simulink model "InvK_Decoupling_Approach_G18"  (R2016a)
settings: Solver=VariableStepAuto  SolverMode=SingleTasking  StartTime=0.0  StopTime=inf  RelTol=1e-3
libraries: vrlib x7, simulink_extras x6
settings Model: Creator=Ricardo Henriques  LastModifiedBy=Ricardo Henriques
settings DebuggingCC: SFUnexpectedBacktrackingDiag=error  SFNoUnconditionalDefaultTransitionDiag=error
settings GRTTargetCC: TargetLangStandard=C99 (ISO)  GeneratePreprocessorConditionals=Use local settings
settings ConfigComp: CovMetricSettings=dwe  CovHtmlReporting=off  CovSaveCumulativeToWorkspaceVar=off  CovSaveSingleToWorkspaceVar=off  CovExternalEMLEnable=on

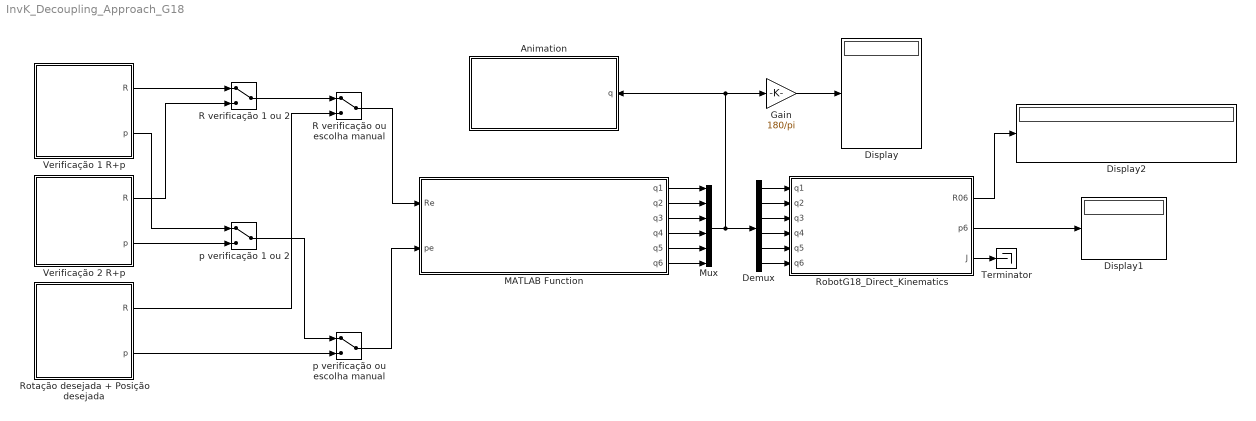
== system InvK_Decoupling_Approach_G18 ==
  "Animation " : Subsystem
  Demux : Demux  Outputs=6
  Display : Display
  Display1 : Display
  Display2 : Display
  Gain : Gain  Gain=180/pi
  MATLAB Function : MATLAB Function  TreatAsAtomicUnit=on
  Mux : Mux  Inputs=6
  R verificação 1 ou 2 : ManualSwitch
  R verificação ou escolha manual : ManualSwitch
  RobotG18_Direct_Kinematics : MATLAB Function  TreatAsAtomicUnit=on
  Rotação desejada + Posição desejada : Subsystem  mask{px=0.663, py=-0.109, pz=0.051, phi=0, theta=-180.0, psi=90}
  Terminator : Terminator
  Verificação 1 R+p : Subsystem
  Verificação 2 R+p : Subsystem
  p verificação 1 ou 2 : ManualSwitch
  p verificação ou escolha manual : ManualSwitch
  wires:
  MATLAB Function/1(q1) -> Mux/1
  MATLAB Function/2(q2) -> Mux/2
  MATLAB Function/6(q6) -> Mux/6
  MATLAB Function/5(q5) -> Mux/5
  MATLAB Function/4(q4) -> Mux/4
  MATLAB Function/3(q3) -> Mux/3
  Mux/1 -> "Animation "/1("q "), Gain/1, Demux/1
  Demux/1 -> RobotG18_Direct_Kinematics/1(q1)
  Demux/2 -> RobotG18_Direct_Kinematics/2(q2)
  Demux/3 -> RobotG18_Direct_Kinematics/3(q3)
  Demux/4 -> RobotG18_Direct_Kinematics/4(q4)
  Demux/5 -> RobotG18_Direct_Kinematics/5(q5)
  Demux/6 -> RobotG18_Direct_Kinematics/6(q6)
  RobotG18_Direct_Kinematics/3(J) -> Terminator/1
  RobotG18_Direct_Kinematics/2(p6) -> Display1/1
  RobotG18_Direct_Kinematics/1(R06) -> Display2/1
  Gain/1 -> Display/1
  R verificação ou escolha manual/1 -> MATLAB Function/1(Re)
  p verificação ou escolha manual/1 -> MATLAB Function/2(pe)
  R verificação 1 ou 2/1 -> R verificação ou escolha manual/1
  p verificação 1 ou 2/1 -> p verificação ou escolha manual/1
  Rotação desejada + Posição desejada/1(R) -> R verificação ou escolha manual/2
  Rotação desejada + Posição desejada/2(p) -> p verificação ou escolha manual/2
  Verificação 1 R+p/1(R) -> R verificação 1 ou 2/1
  Verificação 2 R+p/1(R) -> R verificação 1 ou 2/2
  Verificação 2 R+p/2(p) -> p verificação 1 ou 2/2
  Verificação 1 R+p/2(p) -> p verificação 1 ou 2/1

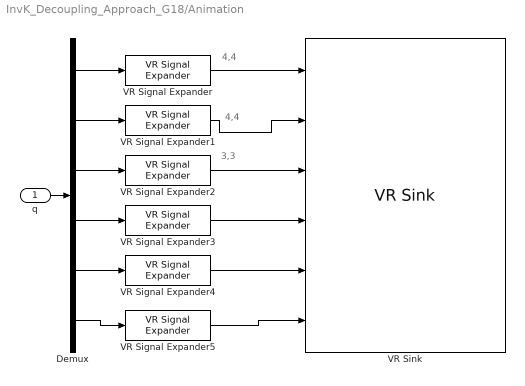
== system InvK_Decoupling_Approach_G18/Animation  ==
  note: 4,4
  note: 3,3
  note: 4,4
  "q " : Inport
  Demux : Demux  Outputs=6
  VR Signal Expander{,1..5} (6 alike) : vrlib/VR Signal Expander  outwidth=4  outidx=4
  VR Sink : vrlib/VR Sink  InstantiateOnLoad=on  SampleTime=0.1  ViewEnable=on  RemoteChange=off  RemoteView=off  FieldsWritten=Jt1_DH_dv.rotation.4.1.1.double#Jt2_DH_dv.rotation.4.1.1.double#Jt3_DH_dv.rotation.4.1.1.double#Jt4_DH_dv.rotation.4.1.1.double#Jt5_DH_dv.rotation.4.1.1.double#Jt6_DH_dv.rotation.4.1.1.double  WorldFileName=RobotG18_Opt_NoAxes.wrl  WorldDescription=D-H Reference Frames for Virtual Reality Robot  AutoView=off  VideoDimensions=[]  AllowVariableSize=off
  wires:
  "q "/1 -> Demux/1
  Demux/1 -> VR Signal Expander/1
  Demux/2 -> VR Signal Expander1/1
  Demux/3 -> VR Signal Expander2/1
  Demux/4 -> VR Signal Expander3/1
  Demux/5 -> VR Signal Expander4/1
  Demux/6 -> VR Signal Expander5/1
  VR Signal Expander/1 -> VR Sink/1
  VR Signal Expander1/1 -> VR Sink/2
  VR Signal Expander5/1 -> VR Sink/6
  VR Signal Expander2/1 -> VR Sink/3
  VR Signal Expander3/1 -> VR Sink/4
  VR Signal Expander4/1 -> VR Sink/5

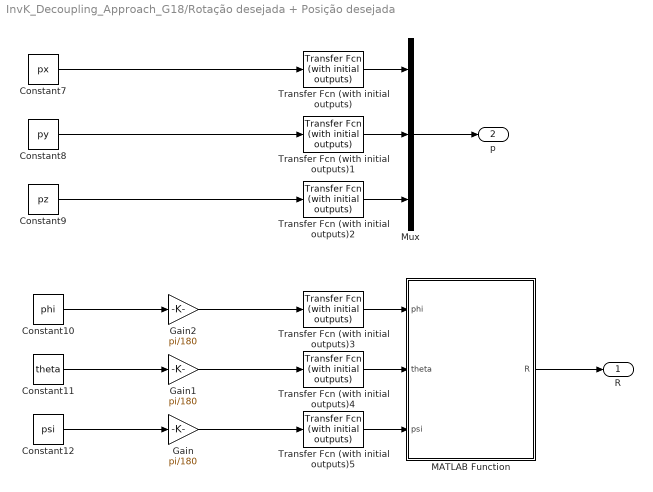
== system InvK_Decoupling_Approach_G18/Rotação desejada + Posição desejada ==
  Constant10 : Constant  Value=phi
  Constant11 : Constant  Value=theta
  Constant12 : Constant  Value=psi
  Constant7 : Constant  Value=px
  Constant8 : Constant  Value=py
  Constant9 : Constant  Value=pz
  Gain : Gain  Gain=pi/180
  Gain1 : Gain  Gain=pi/180
  Gain2 : Gain  Gain=pi/180
  MATLAB Function : MATLAB Function  TreatAsAtomicUnit=on
  Mux : Mux  Inputs=3
  Transfer Fcn (with initial outputs) : simulink_extras/Additional Linear/Transfer Fcn (with initial outputs)  N=[2]  D="[1  2]"  Y0=px  U0=0
  Transfer Fcn (with initial outputs)1 : simulink_extras/Additional Linear/Transfer Fcn (with initial outputs)  N=[2]  D="[1  2]"  Y0=py  U0=0
  Transfer Fcn (with initial outputs)2 : simulink_extras/Additional Linear/Transfer Fcn (with initial outputs)  N=[2]  D="[1  2]"  Y0=pz  U0=0
  Transfer Fcn (with initial outputs)3 : simulink_extras/Additional Linear/Transfer Fcn (with initial outputs)  N=[2]  D="[1  2]"  Y0=phi  U0=0
  Transfer Fcn (with initial outputs)4 : simulink_extras/Additional Linear/Transfer Fcn (with initial outputs)  N=[2]  D="[1  2]"  Y0=theta  U0=0
  Transfer Fcn (with initial outputs)5 : simulink_extras/Additional Linear/Transfer Fcn (with initial outputs)  N=[2]  D="[1  2]"  Y0=psi  U0=0
  R : Outport
  p : Outport  Port=2
  wires:
  Constant8/1 -> Transfer Fcn (with initial outputs)1/1
  Constant9/1 -> Transfer Fcn (with initial outputs)2/1
  Constant12/1 -> Gain/1
  Constant7/1 -> Transfer Fcn (with initial outputs)/1
  Constant11/1 -> Gain1/1
  Constant10/1 -> Gain2/1
  Transfer Fcn (with initial outputs)5/1 -> MATLAB Function/3(psi)
  Transfer Fcn (with initial outputs)3/1 -> MATLAB Function/1(phi)
  Transfer Fcn (with initial outputs)4/1 -> MATLAB Function/2(theta)
  Transfer Fcn (with initial outputs)/1 -> Mux/1
  Transfer Fcn (with initial outputs)1/1 -> Mux/2
  Transfer Fcn (with initial outputs)2/1 -> Mux/3
  Gain2/1 -> Transfer Fcn (with initial outputs)3/1
  Gain1/1 -> Transfer Fcn (with initial outputs)4/1
  Gain/1 -> Transfer Fcn (with initial outputs)5/1
  Mux/1 -> p/1
  MATLAB Function/1(R) -> R/1

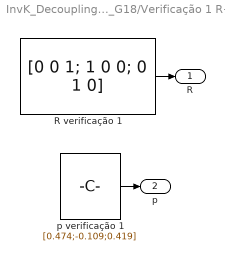
== system InvK_Decoupling_Approach_G18/Verificação 1 R+p ==
  R verificação 1 : Constant  Value=[0 0 1; 1 0 0; 0 1 0]  VectorParams1D=off
  p verificação 1 : Constant  Value=[0.474;-0.109;0.419]  VectorParams1D=off
  R : Outport
  p : Outport  Port=2
  wires:
  p verificação 1/1 -> p/1
  R verificação 1/1 -> R/1

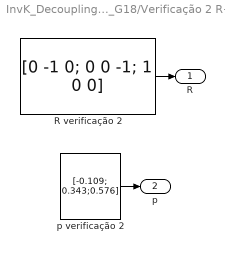
== system InvK_Decoupling_Approach_G18/Verificação 2 R+p ==
  R verificação 2 : Constant  Value=[0 -1 0; 0 0 -1; 1 0 0]  VectorParams1D=off
  p verificação 2 : Constant  Value=[-0.109; 0.343;0.576]  VectorParams1D=off
  R : Outport
  p : Outport  Port=2
  wires:
  p verificação 2/1 -> p/1
  R verificação 2/1 -> R/1

== matlab function InvK_Decoupling_Approach_G18/RobotG18_Direct_Kinematics ==
  data: q1 input; R06 output; q2 input; q3 input; q4 input; q5 input; q6 input; p6 output; J output
function [R06,p6,J] = RobotG18_Direct_Kinematics(q1,q2,q3,q4,q5,q6)
%#codegen

%    This function was generated by the Symbolic Math Toolbox version 7.0.
%    15-Apr-2021 18:49:51

t2 = q2+q3+q4;
t3 = cos(q1);
t4 = sin(q6);
t5 = sin(q1);
t6 = sin(q5);
t7 = t5.*t6;
t8 = cos(t2);
t9 = cos(q5);
t10 = t7-t3.*t8.*t9;
t11 = sin(t2);
t12 = cos(q6);
t13 = t3.*t6;
t14 = t5.*t8.*t9;
t15 = t13+t14;
t16 = q2+q3;
t17 = cos(q2);
t18 = sin(q2);
t19 = sin(q3);
t20 = cos(t16);
t21 = sin(q4);
t22 = sin(t16);
t23 = cos(q4);
t24 = cos(q3);
t25 = t5.*t17.*(1.7e1./4.0e1);
t26 = t5.*t6.*t8.*(4.1e1./5.0e2);
t27 = t5.*t17.*t24.*(4.9e1./1.25e2);
t28 = t22.*(4.9e1./1.25e2);
t29 = t18.*(1.7e1./4.0e1);
t30 = t20.*t21.*(4.1e1./5.0e2);
t31 = t22.*t23.*(4.1e1./5.0e2);
t32 = t30+t31;
t33 = t6.*t32;
t34 = t20.*t23.*(1.9e1./2.0e2);
t35 = t8.*(1.9e1./2.0e2);
t36 = t6.*t11.*(4.1e1./5.0e2);
t37 = t5.*(1.09e2./1.0e3);
t38 = t3.*t17.*(1.7e1./4.0e1);
t39 = t5.*t9.*(4.1e1./5.0e2);
t40 = t3.*t6.*t8.*(4.1e1./5.0e2);
t41 = t3.*t17.*t24.*(4.9e1./1.25e2);
t42 = t37+t38+t39+t40+t41-t3.*t18.*t19.*(4.9e1./1.25e2)-t3.*t20.*t21.*(1.9e1./2.0e2)-t3.*t22.*t23.*(1.9e1./2.0e2);
t43 = t28+t29+t33+t34-t21.*t22.*(1.9e1./2.0e2);
t44 = t28+t35+t36;
t45 = t35+t36;
t46 = q2+q3+q4+q5;
t47 = sin(t46);
t48 = t47.*(4.1e1./1.0e3);
t49 = t20.*(4.9e1./1.25e2);
t50 = q2+q3+q4-q5;
t51 = sin(t50);
t52 = t5.*t9;
t53 = t3.*t6.*t8;
t54 = t52+t53;
t55 = t5.*t6.*t8;
t56 = t55-t3.*t9;
t57 = t6.*t11;
R06 = reshape([-t10.*t12-t3.*t4.*t11,t12.*t15-t4.*t5.*t11,t4.*t8+t9.*t11.*t12,t4.*t10-t3.*t11.*t12,-t4.*t15-t5.*t11.*t12,t8.*t12-t4.*t9.*t11,t54,t56,t57],[3,3]);
if nargout > 1
    p6 = [t42;t3.*(-1.09e2./1.0e3)+t25+t26+t27-t3.*t9.*(4.1e1./5.0e2)-t5.*t18.*t19.*(4.9e1./1.25e2)-t5.*t20.*t21.*(1.9e1./2.0e2)-t5.*t22.*t23.*(1.9e1./2.0e2);t28+t29+t33+t34-t21.*t22.*(1.9e1./2.0e2)+8.9e1./1.0e3];
end
if nargout > 2
    J = reshape([t3.*(1.09e2./1.0e3)-t25-t26-t27+t3.*t9.*(4.1e1./5.0e2)+t5.*t18.*t19.*(4.9e1./1.25e2)+t5.*t20.*t21.*(1.9e1./2.0e2)+t5.*t22.*t23.*(1.9e1./2.0e2),t42,0.0,0.0,0.0,1.0,-t3.*t43,-t5.*t43,t11.*(-1.9e1./2.0e2)+t17.*(1.7e1./4.0e1)+t48+t49-t51.*(4.1e1./1.0e3),t5,-t3,0.0,-t3.*t44,-t5.*t44,t11.*(-1.9e1./2.0e2)+t48+t49-t51.*(4.1e1./1.0e3),t5,-t3,0.0,-t3.*t45,-t5.*t45,t11.*(-1.9e1./2.0e2)+t48-t51.*(4.1e1./1.0e3),t5,-t3,0.0,t5.*t6.*(-4.1e1./5.0e2)-t3.*t9.*t17.*t19.*t21.*(4.1e1./5.0e2)-t3.*t9.*t18.*t19.*t23.*(4.1e1./5.0e2)-t3.*t9.*t18.*t21.*t24.*(4.1e1./5.0e2)+t3.*t9.*t17.*t23.*t24.*(4.1e1./5.0e2),t3.*t6.*(4.1e1./5.0e2)-t5.*t9.*t17.*t19.*t21.*(4.1e1./5.0e2)-t5.*t9.*t18.*t19.*t23.*(4.1e1./5.0e2)-t5.*t9.*t18.*t21.*t24.*(4.1e1./5.0e2)+t5.*t9.*t17.*t23.*t24.*(4.1e1./5.0e2),t48+t51.*(4.1e1./1.0e3),-t3.*t11,-t5.*t11,t8,0.0,0.0,0.0,t54,t56,t57],[6,6]);
end

== matlab function InvK_Decoupling_Approach_G18/MATLAB Function ==
  data: Re input; q1 output; pe input; q2 output; q3 output; q4 output; q5 output; q6 output
function [q1,q2,q3,q4,q5,q6] = Robot618_Inverse_Kinematics_Decoupling(Re,pe)
% Esta função cálcula os ângulos das juntas de rotação através da abordagem
% do desacoplamento.
%
% Inputs: - Re: Matriz de Rotação entre o referêncial 6 e o referencial 0.
%         - pe: Vetor de posição do referêncial 6 em relação ao referencial 0
%
% Outputs: - q1,q2,q3,q4,q5,q6: ângulos entre os eixos x_i-1 e x_i sobre o
% eixo z_i.
%
% Catarina Pires 90230
% Ricardo Henriques 90349
% Última Edição: 22/04/2021
% ------------------------------------------------------------------------
%Cálculo da Matriz de Transformação Homogénea
A06_v = zeros(4,4);
A06_v(1:3,1:3) = Re;
A06_v(1:3,4) = pe;
A06_v(4,4) = 1;
d4 = 0.109;
d6 = 0.082;
a2 = 0.425;
a3 = 0.392;

%Cálculo q1
P05 = A06_v*[0;0;-d6;1] - [0;0;0;1];
P05_xy = sqrt(P05(1).^2 + P05(2).^2);
if pe(2,1)>0
    fi = acos(d4/P05_xy);          %verificar o quadrante 
elseif pe(2,1)==0
    if pe(1,1)<0
        fi = -acos(d4/P05_xy);
    else
        fi = acos(d4/P05_xy);
    end
else
    fi = -acos(d4/P05_xy);
end
qsi = atan2(P05(2),P05(1));
q1 = fi + qsi + pi/2;

%Cálculo q5
P16_z = pe(1)*sin(q1) - pe(2)*cos(q1);

if Re(3,1)>0 && Re(3,1)<=1
    q5 = acos((P16_z - d4)/d6);     %verificar o quadrante 
else
    q5 = -acos((P16_z - d4)/d6);
end

%Cálculo q6
DH_6 = [ 0.089    q1    0    pi/2    0; %    'R';
    0        0  0.425    0     0; %    'R';
    0        0  0.392    0     0; %    'R';
    0.109    0    0   -pi/2    0; %    'R';
    0.095    q5    0    pi/2    0; %    'R';
    0.082    0    0     0      0];%    'R'];
p = DH_6(1,1:5);
A01 =[cos(p(2)) -sin(p(2))*cos(p(4))  sin(p(2))*sin(p(4)) p(3)*cos(p(2));
    sin(p(2))  cos(p(2))*cos(p(4)) -cos(p(2))*sin(p(4)) p(3)*sin(p(2));
    0          sin(p(4))            cos(p(4))                 p(1)    ;
    0             0                    0                        1     ];
A61 = inv(inv(A01)*A06_v);
R61= A61(1:3,1:3);
q6 = atan2(R61(2,3),R61(1,3));

%Cálculo q3
DH_3 = [ 0.089    q1    0    pi/2    0; %    'R';
    0        0  0.425    0     0; %    'R';
    0        0  0.392    0     0; %    'R';
    0.109    0    0   -pi/2    0; %    'R';
    0.095    q5    0    pi/2    0; %    'R';
    0.082    q6    0     0      0];%    'R'];
p = DH_3(5,1:5);
A45 =[cos(p(2)) -sin(p(2))*cos(p(4))  sin(p(2))*sin(p(4)) p(3)*cos(p(2));
    sin(p(2))  cos(p(2))*cos(p(4)) -cos(p(2))*sin(p(4)) p(3)*sin(p(2));
    0          sin(p(4))            cos(p(4))                 p(1)    ;
    0             0                    0                        1     ];
p = DH_3(6,1:5);
A56 =[cos(p(2)) -sin(p(2))*cos(p(4))  sin(p(2))*sin(p(4)) p(3)*cos(p(2));
    sin(p(2))  cos(p(2))*cos(p(4)) -cos(p(2))*sin(p(4)) p(3)*sin(p(2));
    0          sin(p(4))            cos(p(4))                 p(1)    ;
    0             0                    0                        1     ];
A14 = inv(A61)*inv(A45*A56);
P13 = A14*[0;d4;0;1] - [0;0;0;1];
q3 = -acos((norm(P13).^2 - a2^2 - a3^2)/(2*a2*a3));

%Cálculo q2
q2 = atan2(P13(2),(P13(1))) - asin((a3*sin(q3)/norm(P13)));

%Cálculo q4
DH_4 = [ 0.089    q1    0    pi/2    0; %    'R';
    0       q2  0.425    0     0; %    'R';
    0       q3  0.392    0     0; %    'R';
    0.109    0    0   -pi/2    0; %    'R';
    0.095    q5    0    pi/2    0; %    'R';
    0.082    q6    0     0      0];%    'R'];
p = DH_4(2,1:5);
A12 =[cos(p(2)) -sin(p(2))*cos(p(4))  sin(p(2))*sin(p(4)) p(3)*cos(p(2));
    sin(p(2))  cos(p(2))*cos(p(4)) -cos(p(2))*sin(p(4)) p(3)*sin(p(2));
    0          sin(p(4))            cos(p(4))                 p(1)    ;
    0             0                    0                        1     ];
p = DH_4(3,1:5);
A23 =[cos(p(2)) -sin(p(2))*cos(p(4))  sin(p(2))*sin(p(4)) p(3)*cos(p(2));
    sin(p(2))  cos(p(2))*cos(p(4)) -cos(p(2))*sin(p(4)) p(3)*sin(p(2));
    0          sin(p(4))            cos(p(4))                 p(1)    ;
    0             0                    0                        1     ];
A34 = inv(A12*A23)*A14;
q4 = atan2(A34(2,1),A34(1,1));

end

== matlab function InvK_Decoupling_Approach_G18/Rotação desejada + Posição desejada/MATLAB Function ==
  data: phi input; R output; theta input; psi input
function R  = matriz_R(phi, theta,psi)

s_x = sin(phi);
s_y = sin(theta);
s_z = sin(psi);

c_x = cos(phi);
c_y = cos(theta);
c_z = cos(psi);
 
R = [(c_x*c_y*c_z)-(s_x*s_z)    -(c_x*c_y*s_z)-(s_x*c_z)  c_x*s_y;
     (s_x*c_y*c_z)+(c_x*s_z)    -(s_x*c_y*s_z)+(c_x*c_z)  s_x*s_y;
     -s_y*c_z                    s_y*s_z                  c_y    ];
end
